simulink model "monitorWrench"  (R2012b)
settings: Solver=FixedStepDiscrete  StartTime=0.0  StopTime=inf  FixedStep=0.01  RelTol=1e-3
libraries: WBCLibrary x3, utility x1
settings Model: Creator=daniele  LastModifiedBy=daniele

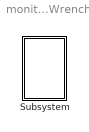
== system monitorWrench ==
  Subsystem : Subsystem  mask{robotName='iCubGenova01', localName='wrenchMonitor', Ts=0.01}

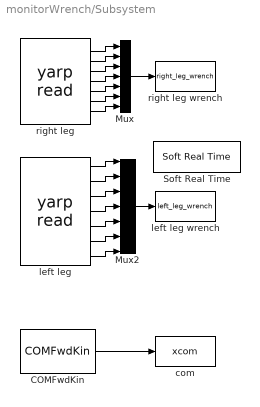
== system monitorWrench/Subsystem ==
  "COMFwdKin " : WBCLibrary/wholeBodyModel/Forward Kinematics/COMFwdKin   robotName=robotName  localName=localName
  Mux : Mux  Inputs=7
  Mux2 : Mux  Inputs=7
  Soft Real Time : utility/Soft Real Time  x=1
  com : ToWorkspace  VariableName=xcom  SampleTime=-1  SaveFormat=Timeseries
  left leg : WBCLibrary/Utilities/yarp read  from=['/wholeBodyDynamicsTree/left_leg/endEffectorWrench:o']  to='...'  num=6  blocking=off  timestamp=on
  left leg wrench : ToWorkspace  VariableName=left_leg_wrench  SampleTime=-1  SaveFormat=Timeseries
  right leg : WBCLibrary/Utilities/yarp read  from='/wholeBodyDynamicsTree/right_leg/endEffectorWrench:o'  to='...'  num=6  blocking=off  timestamp=on
  right leg wrench : ToWorkspace  VariableName=right_leg_wrench  SampleTime=-1  SaveFormat=Timeseries
  wires:
  right leg/2 -> Mux/2
  "COMFwdKin "/1 -> com/1
  right leg/4 -> Mux/4
  Mux/1 -> right leg wrench/1
  right leg/1 -> Mux/1
  right leg/5 -> Mux/5
  right leg/3 -> Mux/3
  right leg/6 -> Mux/6
  left leg/1 -> Mux2/1
  left leg/2 -> Mux2/2
  left leg/3 -> Mux2/3
  left leg/4 -> Mux2/4
  left leg/5 -> Mux2/5
  left leg/6 -> Mux2/6
  Mux2/1 -> left leg wrench/1
  right leg/7 -> Mux/7
  left leg/7 -> Mux2/7
